simulink model "jianmo_1and2"  (R2020b)
settings: Solver=VariableStepAuto  StartTime=0.0  StopTime=100  RelTol=1e-3
settings Model: Creator=19017  LastModifiedBy=19017

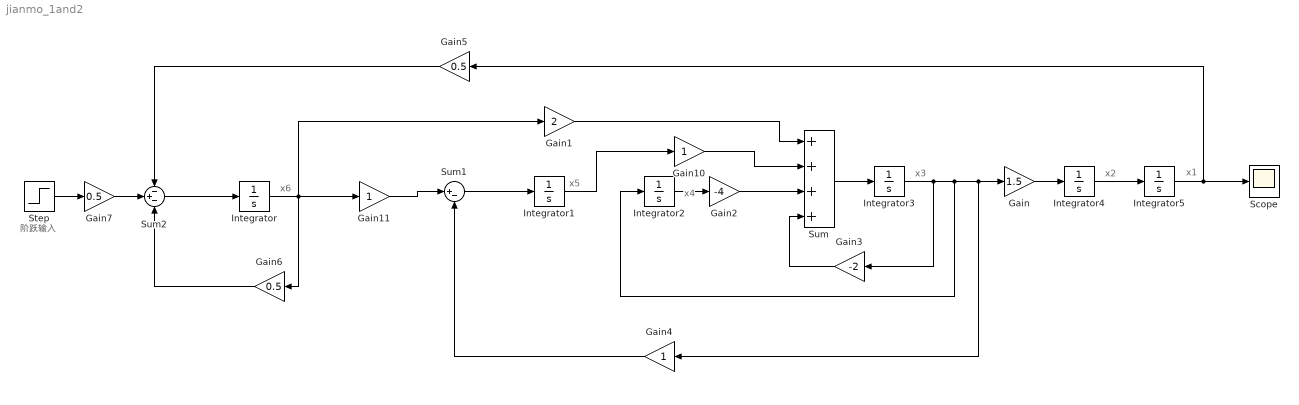
== system jianmo_1and2 ==
  note: 阶跃输入
  note: x1
  note: x2
  note: x3
  note: x4
  note: x5
  note: x6
  Gain : Gain  Gain=1.5
  Gain1 : Gain  Gain=2
  Gain10 : Gain
  Gain11 : Gain
  Gain2 : Gain  Gain=-4
  Gain3 : Gain  Gain=-2
  Gain4 : Gain
  Gain5 : Gain  Gain=0.5
  Gain6 : Gain  Gain=0.5
  Gain7 : Gain  Gain=0.5
  Integrator{,1..5} (6 alike) : Integrator
  Scope : Scope
  Step : Step  SampleTime=0
  Sum : Sum  Inputs=++++
  Sum1 : Sum  Inputs=|+-
  Sum2 : Sum  Inputs=-+-
  wires:
  Integrator4/1 -> Integrator5/1
  Gain/1 -> Integrator4/1
  Integrator2/1 -> Gain2/1
  Integrator3/1 -> Gain3/1, Gain4/1, Gain/1, Integrator2/1
  Sum/1 -> Integrator3/1
  Gain3/1 -> Sum/4
  Gain2/1 -> Sum/3
  Integrator1/1 -> Gain10/1
  Gain10/1 -> Sum/2
  Integrator/1 -> Gain1/1, Gain6/1, Gain11/1
  Gain1/1 -> Sum/1
  Sum1/1 -> Integrator1/1
  Gain11/1 -> Sum1/1
  Gain4/1 -> Sum1/2
  Sum2/1 -> Integrator/1
  Integrator5/1 -> Scope/1, Gain5/1
  Gain5/1 -> Sum2/1
  Gain6/1 -> Sum2/3
  Gain7/1 -> Sum2/2
  Step/1 -> Gain7/1
